simulink model "kinematics_crane"  (R2018b)
settings: Solver=VariableStepAuto  StartTime=0.0  StopTime=Tsim  RelTol=1e-6
model workspace: external: MATLAB File kran_DataFile.m (data not in the file)
undefined symbols (not defined in the file or in its folder): smiData, Ts, X, Y, Z
libraries: sm_lib x99, nesl_utility x28, simulink_extras x2
(part 1 of 3)
settings Model: Creator=Marko  LastModifiedBy=mandicluka
settings SFSimCC: SimCustomHeaderCode="#include \"../temp_cfiles/c_code.h\""  SimParseCustomCode=off
settings SFSimCC: SimUserSources=|
  | ../temp_cfiles/base.c
  | ../temp_cfiles/pulley.c
  | ../temp_cfiles//rot.c
  | ../temp_cfiles/trans1.c
  | ../temp_cfiles/trans2.c
settings SimscapeCC: SimscapeLogType=all  SimscapeLogSimulationStatistics=on  SimscapeLogLimitData=off
settings ExplorerConfigSet: InternalSimMechanicsExplorerSettings="<ExplorerConfiguration><canonicalview>planar_xy</canonicalview><AnimationSetting><BasePlaybackSpeed>1.0</BasePlaybackSpeed><PlaybackSpeedFactor>1.0</PlaybackSpeedFactor></AnimationSetting><TilePanel><TileInfo><Tiles Columns=\"1\" Count=\"1\" Rows=\"1\"><Column Weight=\"1\"/><Row Weight=\"1\"/><Tile Height=\"1\" Width=\"1\" X=\"0\" Y=\"0\"/></Tiles></TileInfo><SceneInfo><SceneViewer><BGColor><R>0.60000002384185791</R><G>0.60000002384185791</G><B>0.60000002384185791</B></BGColor><Camera><DoPerspective>off</DoPerspective><Position><X>10.1383469879859511</X><Y>3.51643315137439361</Y><Z>-1.36564695488922516</Z></Position><Center><X>1.28157942243814538</X><Y>3.51643315137439361</Y><Z>-1.36564695488922516</Z></Center><Up><X>0</X><Y>1</Y><Z>0</Z></Up><ViewLimDist>1</ViewLimDist><YLim>6.81084416950491534</YLim><XLim>4.8510498406429976</XLim></Camera></SceneViewer></SceneInfo></TilePanel><MechEditorPanel><Cameras/><GfxPanelCameraMap/><VideoCreator><PlaybackSpeedRatio>1.0</PlaybackSpeedRatio><FrameRate>30</FrameRate><VideoFormat>Motion JPEG AVI</VideoFormat><FrameSize>auto</FrameSize></VideoCreator></MechEditorPanel></ExplorerConfiguration>"

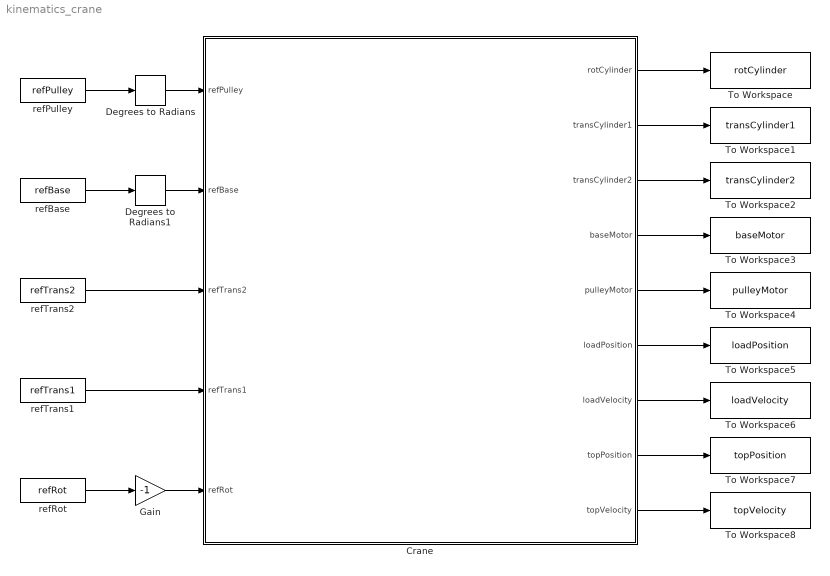
== system kinematics_crane ==
  Crane : Subsystem
  Degrees to Radians : simulink_extras/Transformations/Degrees to Radians
  Degrees to Radians1 : simulink_extras/Transformations/Degrees to Radians
  Gain : Gain  Gain=-1
  To Workspace : ToWorkspace  VariableName=rotCylinder  SaveFormat=Structure With Time  SampleTime=Ts
  To Workspace1 : ToWorkspace  VariableName=transCylinder1  SaveFormat=Structure With Time  SampleTime=Ts
  To Workspace2 : ToWorkspace  VariableName=transCylinder2  SaveFormat=Structure With Time  SampleTime=Ts
  To Workspace3 : ToWorkspace  VariableName=baseMotor  SaveFormat=Structure With Time  SampleTime=Ts
  To Workspace4 : ToWorkspace  VariableName=pulleyMotor  SaveFormat=Structure With Time  SampleTime=Ts
  To Workspace5 : ToWorkspace  VariableName=loadPosition  SaveFormat=Structure With Time  SampleTime=Ts
  To Workspace6 : ToWorkspace  VariableName=loadVelocity  SaveFormat=Structure With Time  SampleTime=Ts
  To Workspace7 : ToWorkspace  VariableName=topPosition  SaveFormat=Structure With Time  SampleTime=Ts
  To Workspace8 : ToWorkspace  VariableName=topVelocity  SaveFormat=Structure With Time  SampleTime=Ts
  refBase : FromWorkspace  VariableName=refBase  SampleTime=0  OutputAfterFinalValue=Holding final value
  refPulley : FromWorkspace  VariableName=refPulley  SampleTime=0  OutputAfterFinalValue=Holding final value
  refRot : FromWorkspace  VariableName=refRot  SampleTime=0  OutputAfterFinalValue=Holding final value
  refTrans1 : FromWorkspace  VariableName=refTrans1  SampleTime=0  OutputAfterFinalValue=Holding final value
  refTrans2 : FromWorkspace  VariableName=refTrans2  SampleTime=0  OutputAfterFinalValue=Holding final value
  wires:
  Crane/1(rotCylinder) -> To Workspace/1
  Crane/2(transCylinder1) -> To Workspace1/1
  Crane/3(transCylinder2) -> To Workspace2/1
  Crane/4(baseMotor) -> To Workspace3/1
  Crane/5(pulleyMotor) -> To Workspace4/1
  Crane/6(loadPosition) -> To Workspace5/1
  Crane/7(loadVelocity) -> To Workspace6/1
  Crane/8(topPosition) -> To Workspace7/1
  Crane/9(topVelocity) -> To Workspace8/1
  refPulley/1 -> Degrees to Radians/1
  refBase/1 -> Degrees to Radians1/1
  refTrans2/1 -> Crane/3(refTrans2)
  refTrans1/1 -> Crane/4(refTrans1)
  refRot/1 -> Gain/1
  Degrees to Radians/1 -> Crane/1(refPulley)
  Degrees to Radians1/1 -> Crane/2(refBase)
  Gain/1 -> Crane/5(refRot)

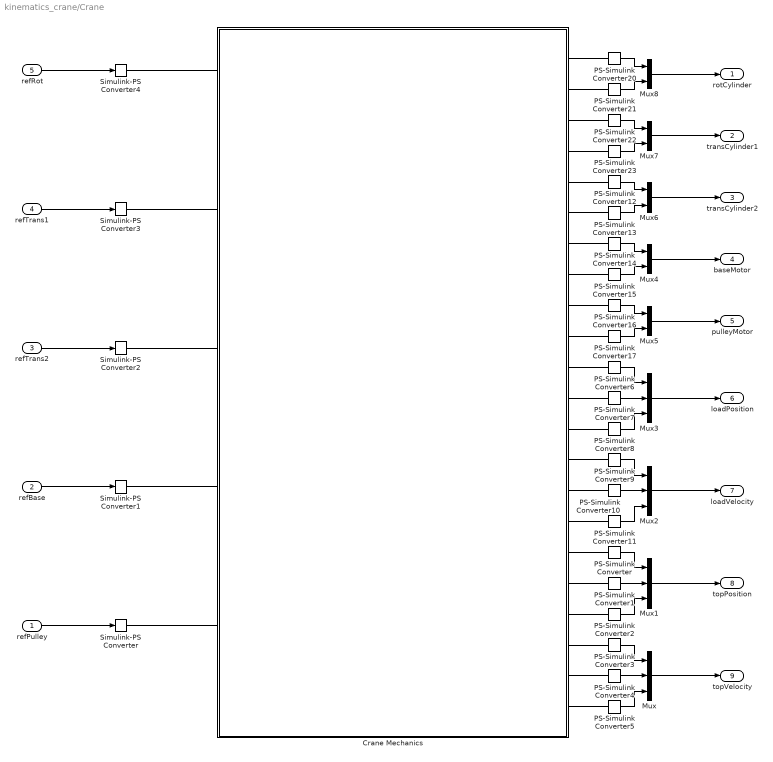
== system kinematics_crane/Crane ==
  refPulley : Inport
  refBase : Inport  Port=2
  refTrans2 : Inport  Port=3
  refTrans1 : Inport  Port=4
  refRot : Inport  Port=5
  Crane Mechanics : Subsystem
  Mux{,1..3} (4 alike) : Mux  Inputs=3
  Mux{4..8} (5 alike) : Mux  Inputs=2
  PS-Simulink Converter{,1..17,20..23} (22 alike) : nesl_utility/PS-Simulink Converter  PhysicalDomain=network_engine_domain  SubClassName=ps_output  LeftPortType=input  RightPortType=output  PseudoPeriodic=off  Frequencies=[]  Unit=1  AffineConversion=off
  Simulink-PS Converter{,1..4} (5 alike) : nesl_utility/Simulink-PS Converter  PhysicalDomain=network_engine_domain  SubClassName=ps_input  LeftPortType=input  RightPortType=output  PseudoPeriodic=off  Frequencies=[]  NoiseDistribution=none  NoiseParameters=[]  Unit=1  AffineConversion=off  FilteringAndDerivatives=filter  SimscapeFilterOrder=2  InputFilterTimeConstant=0.001  UdotUserProvided=0
  rotCylinder : Outport
  transCylinder1 : Outport  Port=2
  transCylinder2 : Outport  Port=3
  baseMotor : Outport  Port=4
  pulleyMotor : Outport  Port=5
  loadPosition : Outport  Port=6
  loadVelocity : Outport  Port=7
  topPosition : Outport  Port=8
  topVelocity : Outport  Port=9
  wires:
  PS-Simulink Converter12/1 -> Mux6/1
  Mux2/1 -> loadVelocity/1
  PS-Simulink Converter11/1 -> Mux2/3
  PS-Simulink Converter22/1 -> Mux7/1
  Mux3/1 -> loadPosition/1
  PS-Simulink Converter4/1 -> Mux/2
  PS-Simulink Converter17/1 -> Mux5/2
  PS-Simulink Converter15/1 -> Mux4/2
  PS-Simulink Converter1/1 -> Mux1/2
  PS-Simulink Converter/1 -> Mux1/1
  PS-Simulink Converter21/1 -> Mux8/2
  PS-Simulink Converter9/1 -> Mux2/1
  PS-Simulink Converter8/1 -> Mux3/3
  PS-Simulink Converter10/1 -> Mux2/2
  PS-Simulink Converter6/1 -> Mux3/1
  PS-Simulink Converter14/1 -> Mux4/1
  PS-Simulink Converter13/1 -> Mux6/2
  Mux6/1 -> transCylinder2/1
  PS-Simulink Converter16/1 -> Mux5/1
  PS-Simulink Converter3/1 -> Mux/1
  PS-Simulink Converter20/1 -> Mux8/1
  PS-Simulink Converter23/1 -> Mux7/2
  Mux1/1 -> topPosition/1
  PS-Simulink Converter5/1 -> Mux/3
  PS-Simulink Converter2/1 -> Mux1/3
  PS-Simulink Converter7/1 -> Mux3/2
  Mux7/1 -> transCylinder1/1
  Mux4/1 -> baseMotor/1
  Mux/1 -> topVelocity/1
  Mux5/1 -> pulleyMotor/1
  Mux8/1 -> rotCylinder/1
  refPulley/1 -> Simulink-PS Converter/1
  refBase/1 -> Simulink-PS Converter1/1
  refTrans2/1 -> Simulink-PS Converter2/1
  refTrans1/1 -> Simulink-PS Converter3/1
  refRot/1 -> Simulink-PS Converter4/1
  connections:
  Crane Mechanics/RConn5 -- PS-Simulink Converter12/LConn1
  Crane Mechanics/RConn7 -- PS-Simulink Converter14/LConn1
  Crane Mechanics/RConn14 -- PS-Simulink Converter9/LConn1
  Crane Mechanics/RConn6 -- PS-Simulink Converter13/LConn1
  Crane Mechanics/RConn15 -- PS-Simulink Converter10/LConn1
  Crane Mechanics/RConn9 -- PS-Simulink Converter16/LConn1
  PS-Simulink Converter2/LConn1 -- Crane Mechanics/RConn19
  Crane Mechanics/RConn16 -- PS-Simulink Converter11/LConn1
  Crane Mechanics/RConn11 -- PS-Simulink Converter6/LConn1
  PS-Simulink Converter5/LConn1 -- Crane Mechanics/RConn22
  Crane Mechanics/RConn4 -- PS-Simulink Converter23/LConn1
  Crane Mechanics/RConn13 -- PS-Simulink Converter8/LConn1
  PS-Simulink Converter/LConn1 -- Crane Mechanics/RConn17
  Crane Mechanics/RConn3 -- PS-Simulink Converter22/LConn1
  Crane Mechanics/RConn8 -- PS-Simulink Converter15/LConn1
  PS-Simulink Converter4/LConn1 -- Crane Mechanics/RConn21
  Crane Mechanics/RConn2 -- PS-Simulink Converter21/LConn1
  Crane Mechanics/RConn12 -- PS-Simulink Converter7/LConn1
  Crane Mechanics/RConn1 -- PS-Simulink Converter20/LConn1
  PS-Simulink Converter1/LConn1 -- Crane Mechanics/RConn18
  Crane Mechanics/RConn10 -- PS-Simulink Converter17/LConn1
  PS-Simulink Converter3/LConn1 -- Crane Mechanics/RConn20
  Simulink-PS Converter/RConn1 -- Crane Mechanics/LConn9
  Crane Mechanics/LConn7 -- Simulink-PS Converter1/RConn1
  Crane Mechanics/LConn5 -- Simulink-PS Converter2/RConn1
  Crane Mechanics/LConn3 -- Simulink-PS Converter3/RConn1
  Crane Mechanics/LConn1 -- Simulink-PS Converter4/RConn1

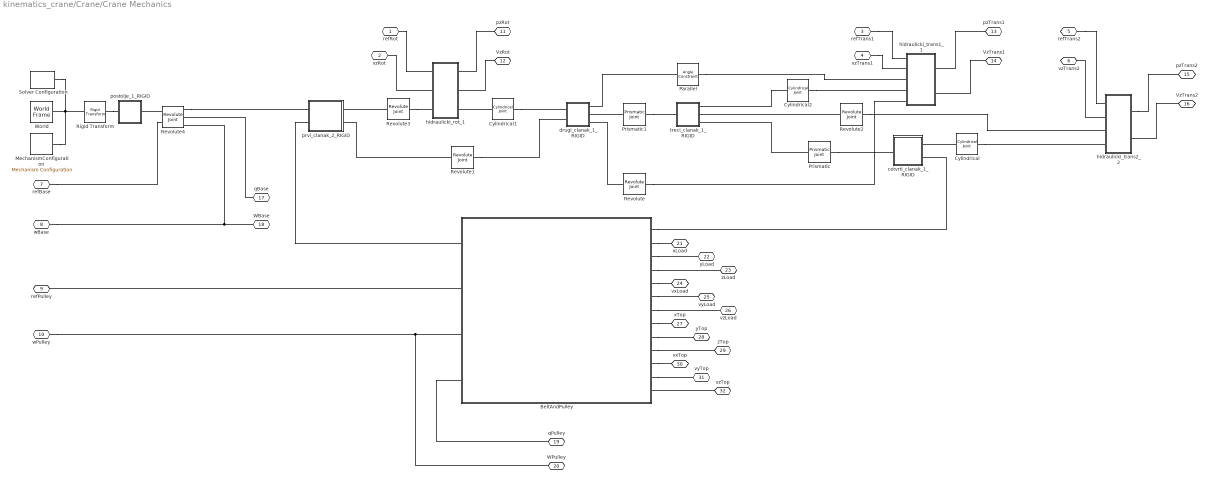
== system kinematics_crane/Crane/Crane Mechanics ==
  BeltAndPulley : Subsystem
  Cylindrical : sm_lib/Joints/Cylindrical Joint  SenseConstraintForce=off  SenseConstraintForceX=off  SenseConstraintForceY=off  SenseConstraintForceZ=off  SenseConstraintTorque=off  SenseConstraintTorqueX=off  SenseConstraintTorqueY=off  SenseConstraintTorqueZ=off  SenseTotalForce=off  SenseTotalForceX=off  SenseTotalForceY=off  SenseTotalForceZ=off  SenseTotalTorque=off  SenseTotalTorqueX=off  SenseTotalTorqueY=off  SenseTotalTorqueZ=off  CompositeWrenchDir=FollowerOnBase  CompositeWrenchFrame=BaseFrame  PzEquilibriumPosition=0  PzEquilibriumPositionUnits=m  PzSpringStiffness=0  PzSpringStiffnessUnits=N/m  PzDampingCoefficient=0  PzDampingCoefficientUnits=N/(m/s)  PzTorqueActuationMode=NoTorque  PzMotionActuationMode=ComputedMotion  PzSensePosition=off  PzSenseVelocity=off  PzSenseAcceleration=off  PzSenseTorqueForce=off  PzPositionTargetSpecify=off  PzPositionTargetPriority=High  PzPositionTargetValue=0  PzPositionTargetValueUnits=m  PzVelocityTargetSpecify=off  PzVelocityTargetPriority=High  PzVelocityTargetValue=0  PzVelocityTargetValueUnits=m/s  RzEquilibriumPosition=0  RzEquilibriumPositionUnits=rad  RzSpringStiffness=0  RzSpringStiffnessUnits=N*m/rad  RzDampingCoefficient=0  RzDampingCoefficientUnits=N*m/(rad/s)  RzTorqueActuationMode=NoTorque  RzMotionActuationMode=ComputedMotion  RzSensePosition=off  RzSenseVelocity=off  RzSenseAcceleration=off  RzSenseTorqueForce=off  RzPositionTargetSpecify=off  RzPositionTargetPriority=High  RzPositionTargetValue=0  RzPositionTargetValueUnits=deg  RzVelocityTargetSpecify=off  RzVelocityTargetPriority=High  RzVelocityTargetValue=0  RzVelocityTargetValueUnits=deg/s
  Cylindrical1 : sm_lib/Joints/Cylindrical Joint  SenseConstraintForce=off  SenseConstraintForceX=off  SenseConstraintForceY=off  SenseConstraintForceZ=off  SenseConstraintTorque=off  SenseConstraintTorqueX=off  SenseConstraintTorqueY=off  SenseConstraintTorqueZ=off  SenseTotalForce=off  SenseTotalForceX=off  SenseTotalForceY=off  SenseTotalForceZ=off  SenseTotalTorque=off  SenseTotalTorqueX=off  SenseTotalTorqueY=off  SenseTotalTorqueZ=off  CompositeWrenchDir=FollowerOnBase  CompositeWrenchFrame=BaseFrame  PzEquilibriumPosition=0  PzEquilibriumPositionUnits=m  PzSpringStiffness=0  PzSpringStiffnessUnits=N/m  PzDampingCoefficient=0  PzDampingCoefficientUnits=N/(m/s)  PzTorqueActuationMode=NoTorque  PzMotionActuationMode=ComputedMotion  PzSensePosition=off  PzSenseVelocity=off  PzSenseAcceleration=off  PzSenseTorqueForce=off  PzPositionTargetSpecify=off  PzPositionTargetPriority=High  PzPositionTargetValue=0  PzPositionTargetValueUnits=m  PzVelocityTargetSpecify=off  PzVelocityTargetPriority=High  PzVelocityTargetValue=0  PzVelocityTargetValueUnits=m/s  RzEquilibriumPosition=0  RzEquilibriumPositionUnits=rad  RzSpringStiffness=0  RzSpringStiffnessUnits=N*m/rad  RzDampingCoefficient=0  RzDampingCoefficientUnits=N*m/(rad/s)  RzTorqueActuationMode=NoTorque  RzMotionActuationMode=ComputedMotion  RzSensePosition=off  RzSenseVelocity=off  RzSenseAcceleration=off  RzSenseTorqueForce=off  RzPositionTargetSpecify=off  RzPositionTargetPriority=High  RzPositionTargetValue=0  RzPositionTargetValueUnits=deg  RzVelocityTargetSpecify=off  RzVelocityTargetPriority=High  RzVelocityTargetValue=0  RzVelocityTargetValueUnits=deg/s
  Cylindrical2 : sm_lib/Joints/Cylindrical Joint  SenseConstraintForce=off  SenseConstraintForceX=off  SenseConstraintForceY=off  SenseConstraintForceZ=off  SenseConstraintTorque=off  SenseConstraintTorqueX=off  SenseConstraintTorqueY=off  SenseConstraintTorqueZ=off  SenseTotalForce=off  SenseTotalForceX=off  SenseTotalForceY=off  SenseTotalForceZ=off  SenseTotalTorque=off  SenseTotalTorqueX=off  SenseTotalTorqueY=off  SenseTotalTorqueZ=off  CompositeWrenchDir=FollowerOnBase  CompositeWrenchFrame=BaseFrame  PzEquilibriumPosition=0  PzEquilibriumPositionUnits=m  PzSpringStiffness=0  PzSpringStiffnessUnits=N/m  PzDampingCoefficient=0  PzDampingCoefficientUnits=N/(m/s)  PzTorqueActuationMode=NoTorque  PzMotionActuationMode=ComputedMotion  PzSensePosition=off  PzSenseVelocity=off  PzSenseAcceleration=off  PzSenseTorqueForce=off  PzPositionTargetSpecify=off  PzPositionTargetPriority=High  PzPositionTargetValue=0  PzPositionTargetValueUnits=m  PzVelocityTargetSpecify=off  PzVelocityTargetPriority=High  PzVelocityTargetValue=0  PzVelocityTargetValueUnits=m/s  RzEquilibriumPosition=0  RzEquilibriumPositionUnits=rad  RzSpringStiffness=0  RzSpringStiffnessUnits=N*m/rad  RzDampingCoefficient=0  RzDampingCoefficientUnits=N*m/(rad/s)  RzTorqueActuationMode=NoTorque  RzMotionActuationMode=ComputedMotion  RzSensePosition=off  RzSenseVelocity=off  RzSenseAcceleration=off  RzSenseTorqueForce=off  RzPositionTargetSpecify=off  RzPositionTargetPriority=High  RzPositionTargetValue=0  RzPositionTargetValueUnits=deg  RzVelocityTargetSpecify=off  RzVelocityTargetPriority=High  RzVelocityTargetValue=0  RzVelocityTargetValueUnits=deg/s
  MechanismConfiguration : sm_lib/Utilities/Mechanism Configuration  UniformGravity=Constant  GravityVector=[0 -9.80665 0]  GravityUnits=m/s^2  LinearizationDelta=0.001
  Parallel : sm_lib/Constraints/Angle Constraint  ConstraintType=Parallel  Angle=45  AngleUnits=deg  SenseSignedTorqueMagnitude=off  SenseTorque=off  SenseForce=off  WrenchDir=FollowerOnBase  WrenchFrame=BaseFrame
      settings: SourceProductName=Simscape Multibody  SourceProductBaseCode=MS
  Prismatic : sm_lib/Joints/Prismatic Joint  SenseConstraintForce=off  SenseConstraintForceX=off  SenseConstraintForceY=off  SenseConstraintForceZ=off  SenseConstraintTorque=off  SenseConstraintTorqueX=off  SenseConstraintTorqueY=off  SenseConstraintTorqueZ=off  SenseTotalForce=off  SenseTotalForceX=off  SenseTotalForceY=off  SenseTotalForceZ=off  SenseTotalTorque=off  SenseTotalTorqueX=off  SenseTotalTorqueY=off  SenseTotalTorqueZ=off  CompositeWrenchDir=FollowerOnBase  CompositeWrenchFrame=BaseFrame  EquilibriumPosition=0  EquilibriumPositionUnits=m  SpringStiffness=0  SpringStiffnessUnits=N/m  DampingCoefficient=0  DampingCoefficientUnits=N/(m/s)  TorqueActuationMode=NoTorque  MotionActuationMode=ComputedMotion  SensePosition=off  SenseVelocity=off  SenseAcceleration=off  SenseTorqueForce=off  PositionTargetSpecify=on  PositionTargetPriority=Low  PositionTargetValue=smiData.PrismaticJoint(1).Pz.Pos  PositionTargetValueUnits=m  VelocityTargetSpecify=off  VelocityTargetPriority=High  VelocityTargetValue=0  VelocityTargetValueUnits=m/s
  Prismatic1 : sm_lib/Joints/Prismatic Joint  SenseConstraintForce=off  SenseConstraintForceX=off  SenseConstraintForceY=off  SenseConstraintForceZ=off  SenseConstraintTorque=off  SenseConstraintTorqueX=off  SenseConstraintTorqueY=off  SenseConstraintTorqueZ=off  SenseTotalForce=off  SenseTotalForceX=off  SenseTotalForceY=off  SenseTotalForceZ=off  SenseTotalTorque=off  SenseTotalTorqueX=off  SenseTotalTorqueY=off  SenseTotalTorqueZ=off  CompositeWrenchDir=FollowerOnBase  CompositeWrenchFrame=BaseFrame  EquilibriumPosition=0  EquilibriumPositionUnits=m  SpringStiffness=0  SpringStiffnessUnits=N/m  DampingCoefficient=0  DampingCoefficientUnits=N/(m/s)  TorqueActuationMode=NoTorque  MotionActuationMode=ComputedMotion  SensePosition=off  SenseVelocity=off  SenseAcceleration=off  SenseTorqueForce=off  PositionTargetSpecify=on  PositionTargetPriority=Low  PositionTargetValue=smiData.PrismaticJoint(2).Pz.Pos  PositionTargetValueUnits=m  VelocityTargetSpecify=off  VelocityTargetPriority=High  VelocityTargetValue=0  VelocityTargetValueUnits=m/s
  Revolute : sm_lib/Joints/Revolute Joint  SenseConstraintForce=off  SenseConstraintForceX=off  SenseConstraintForceY=off  SenseConstraintForceZ=off  SenseConstraintTorque=off  SenseConstraintTorqueX=off  SenseConstraintTorqueY=off  SenseConstraintTorqueZ=off  SenseTotalForce=off  SenseTotalForceX=off  SenseTotalForceY=off  SenseTotalForceZ=off  SenseTotalTorque=off  SenseTotalTorqueX=off  SenseTotalTorqueY=off  SenseTotalTorqueZ=off  CompositeWrenchDir=FollowerOnBase  CompositeWrenchFrame=BaseFrame  EquilibriumPosition=0  EquilibriumPositionUnits=rad  SpringStiffness=0  SpringStiffnessUnits=N*m/rad  DampingCoefficient=0  DampingCoefficientUnits=N*m/(rad/s)  TorqueActuationMode=NoTorque  MotionActuationMode=ComputedMotion  SensePosition=off  SenseVelocity=off  SenseAcceleration=off  SenseTorqueForce=off  PositionTargetSpecify=on  PositionTargetPriority=Low  PositionTargetValue=smiData.RevoluteJoint(4).Rz.Pos  PositionTargetValueUnits=deg  VelocityTargetSpecify=off  VelocityTargetPriority=High  VelocityTargetValue=0  VelocityTargetValueUnits=deg/s
  Revolute1 : sm_lib/Joints/Revolute Joint  SenseConstraintForce=off  SenseConstraintForceX=off  SenseConstraintForceY=off  SenseConstraintForceZ=off  SenseConstraintTorque=off  SenseConstraintTorqueX=off  SenseConstraintTorqueY=off  SenseConstraintTorqueZ=off  SenseTotalForce=off  SenseTotalForceX=off  SenseTotalForceY=off  SenseTotalForceZ=off  SenseTotalTorque=off  SenseTotalTorqueX=off  SenseTotalTorqueY=off  SenseTotalTorqueZ=off  CompositeWrenchDir=FollowerOnBase  CompositeWrenchFrame=BaseFrame  EquilibriumPosition=0  EquilibriumPositionUnits=rad  SpringStiffness=0  SpringStiffnessUnits=N*m/rad  DampingCoefficient=0  DampingCoefficientUnits=N*m/(rad/s)  TorqueActuationMode=NoTorque  MotionActuationMode=ComputedMotion  SensePosition=off  SenseVelocity=off  SenseAcceleration=off  SenseTorqueForce=off  PositionTargetSpecify=on  PositionTargetPriority=Low  PositionTargetValue=smiData.RevoluteJoint(5).Rz.Pos  PositionTargetValueUnits=deg  VelocityTargetSpecify=off  VelocityTargetPriority=High  VelocityTargetValue=0  VelocityTargetValueUnits=deg/s
  Revolute2 : sm_lib/Joints/Revolute Joint  SenseConstraintForce=off  SenseConstraintForceX=off  SenseConstraintForceY=off  SenseConstraintForceZ=off  SenseConstraintTorque=off  SenseConstraintTorqueX=off  SenseConstraintTorqueY=off  SenseConstraintTorqueZ=off  SenseTotalForce=off  SenseTotalForceX=off  SenseTotalForceY=off  SenseTotalForceZ=off  SenseTotalTorque=off  SenseTotalTorqueX=off  SenseTotalTorqueY=off  SenseTotalTorqueZ=off  CompositeWrenchDir=FollowerOnBase  CompositeWrenchFrame=BaseFrame  EquilibriumPosition=0  EquilibriumPositionUnits=rad  SpringStiffness=0  SpringStiffnessUnits=N*m/rad  DampingCoefficient=0  DampingCoefficientUnits=N*m/(rad/s)  TorqueActuationMode=NoTorque  MotionActuationMode=ComputedMotion  SensePosition=off  SenseVelocity=off  SenseAcceleration=off  SenseTorqueForce=off  PositionTargetSpecify=on  PositionTargetPriority=Low  PositionTargetValue=smiData.RevoluteJoint(6).Rz.Pos  PositionTargetValueUnits=deg  VelocityTargetSpecify=off  VelocityTargetPriority=High  VelocityTargetValue=0  VelocityTargetValueUnits=deg/s
  Revolute3 : sm_lib/Joints/Revolute Joint  SenseConstraintForce=off  SenseConstraintForceX=off  SenseConstraintForceY=off  SenseConstraintForceZ=off  SenseConstraintTorque=off  SenseConstraintTorqueX=off  SenseConstraintTorqueY=off  SenseConstraintTorqueZ=off  SenseTotalForce=off  SenseTotalForceX=off  SenseTotalForceY=off  SenseTotalForceZ=off  SenseTotalTorque=off  SenseTotalTorqueX=off  SenseTotalTorqueY=off  SenseTotalTorqueZ=off  CompositeWrenchDir=FollowerOnBase  CompositeWrenchFrame=BaseFrame  EquilibriumPosition=0  EquilibriumPositionUnits=rad  SpringStiffness=0  SpringStiffnessUnits=N*m/rad  DampingCoefficient=0  DampingCoefficientUnits=N*m/(rad/s)  TorqueActuationMode=NoTorque  MotionActuationMode=ComputedMotion  SensePosition=off  SenseVelocity=off  SenseAcceleration=off  SenseTorqueForce=off  PositionTargetSpecify=on  PositionTargetPriority=Low  PositionTargetValue=smiData.RevoluteJoint(7).Rz.Pos  PositionTargetValueUnits=deg  VelocityTargetSpecify=off  VelocityTargetPriority=High  VelocityTargetValue=0  VelocityTargetValueUnits=deg/s
  Revolute4 : sm_lib/Joints/Revolute Joint  SenseConstraintForce=off  SenseConstraintForceX=off  SenseConstraintForceY=off  SenseConstraintForceZ=off  SenseConstraintTorque=off  SenseConstraintTorqueX=off  SenseConstraintTorqueY=off  SenseConstraintTorqueZ=off  SenseTotalForce=off  SenseTotalForceX=off  SenseTotalForceY=off  SenseTotalForceZ=off  SenseTotalTorque=off  SenseTotalTorqueX=off  SenseTotalTorqueY=off  SenseTotalTorqueZ=off  CompositeWrenchDir=FollowerOnBase  CompositeWrenchFrame=BaseFrame  EquilibriumPosition=0  EquilibriumPositionUnits=rad  SpringStiffness=0  SpringStiffnessUnits=N*m/rad  DampingCoefficient=500  DampingCoefficientUnits=N*m/(rad/s)  TorqueActuationMode=ComputedTorque  MotionActuationMode=InputMotion  SensePosition=on  SenseVelocity=on  SenseAcceleration=off  SenseTorqueForce=off  PositionTargetSpecify=on  PositionTargetPriority=High  PositionTargetValue=0  PositionTargetValueUnits=deg  VelocityTargetSpecify=off  VelocityTargetPriority=High  VelocityTargetValue=0  VelocityTargetValueUnits=deg/s
  Rigid Transform : sm_lib/Frames and Transforms/Rigid Transform  TranslationMethod=Cartesian  TranslationStandardOffset=0  TranslationLengthUnit=m  TranslationStandardAxis=+Z  TranslationCartesianOffset=[0 0.86 0]  TranslationROffset=0  TranslationROffsetUnits=m  TranslationZOffset=0  TranslationZOffsetUnits=m  TranslationThetaOffset=0  TranslationThetaOffsetUnits=deg  RotationMethod=StandardAxis  RotationAngleUnits=deg  RotationStandardAxis=-Y  RotationAngle=90  RotationArbitraryAxis=[0 0 1]  FollAlignAxisA=+X  BaseAlignAxisA=+Y  FollAlignAxisB=+Y  BaseAlignAxisB=+Z  RotationSequenceAxes=FollowerAxes  RotationSequence=XYX  RotationSequenceAngles=[0 0 0]  RotationSequenceAnglesUnits=deg  RotationMatrix=[1 0 0; 0 1 0; 0 0 1]
  Solver Configuration : nesl_utility/Solver Configuration  PhysicalDomain=network_engine_domain  SubClassName=solver  LeftPortType=input  RightPortType=generic  Tones=[]  Harmonics=[]  SimulateNoise=off  Profile=off  UseLocalSampling=off  EnableSwitchedLinearOptims=on  FrequencyDomain=off  UseCCode=off  RelTol=0.001  AbsTol=1e-06  MinStep=1e-09  ToWorkspace=off  RevertToSquareIcSolve=off  NumHomotopyIterations=100  PhasorMode=off  PhasorModeNumHarmonics=1  DoDC=off  ResidualTolerance=1e-09  UseLocalSolver=off  LocalSolverChoice=NE_BACKWARD_EULER_ADVANCER  LocalSolverSampleTime=0.001  DoFixedCost=off  MaxNonlinIter=3  MaxModeIter=2  LinearAlgebra=auto  EquationFormulation=NE_TIME_EF  DelaysMemoryBudget=1024  AutomaticFiltering=on  FilteringTimeConstant=0.0001  PartitionStorageMethod=AS_NEEDED  PartitionMemoryBudget=1024
  World : sm_lib/Frames and Transforms/World Frame
  cetvrti_clanak_1_RIGID : Subsystem
  drugi_clanak_1_RIGID : Subsystem
  hidraulicki_rot_1 : Subsystem
  hidraulicki_trans1_1 : Subsystem
  hidraulicki_trans2_2 : Subsystem
  postolje_1_RIGID : Subsystem
  prvi_clanak_2_RIGID : Subsystem
  treci_clanak_1_RIGID : Subsystem
  refRot : PMIOPort  Side=Left
  vzRot : PMIOPort  Port=2  Side=Left
  refTrans1 : PMIOPort  Port=3  Side=Left
  vzTrans1 : PMIOPort  Port=4  Side=Left
  refTrans2 : PMIOPort  Port=5  Side=Left
  vzTrans2 : PMIOPort  Port=6  Side=Left
  refBase : PMIOPort  Port=7  Side=Left
  wBase : PMIOPort  Port=8  Side=Left
  refPulley : PMIOPort  Port=9  Side=Left
  wPulley : PMIOPort  Port=10  Side=Left
  pzRot : PMIOPort  Port=11  Side=Right
  VzRot : PMIOPort  Port=12  Side=Right
  pzTrans1 : PMIOPort  Port=13  Side=Right
  VzTrans1 : PMIOPort  Port=14  Side=Right
  pzTrans2 : PMIOPort  Port=15  Side=Right
  VzTrans2 : PMIOPort  Port=16  Side=Right
  qBase : PMIOPort  Port=17  Side=Right
  WBase : PMIOPort  Port=18  Side=Right
  qPulley : PMIOPort  Port=19  Side=Right
  WPulley : PMIOPort  Port=20  Side=Right
  xLoad : PMIOPort  Port=21  Side=Right
  yLoad : PMIOPort  Port=22  Side=Right
  zLoad : PMIOPort  Port=23  Side=Right
  vxLoad : PMIOPort  Port=24  Side=Right
  vyLoad : PMIOPort  Port=25  Side=Right
  vzLoad : PMIOPort  Port=26  Side=Right
  xTop : PMIOPort  Port=27  Side=Right
  yTop : PMIOPort  Port=28  Side=Right
  zTop : PMIOPort  Port=29  Side=Right
  vxTop : PMIOPort  Port=30  Side=Right
  vyTop : PMIOPort  Port=31  Side=Right
  vzTop : PMIOPort  Port=32  Side=Right
  connections:
  Cylindrical2/RConn1 -- hidraulicki_trans1_1/LConn4
  MechanismConfiguration/RConn1 -- Solver Configuration/RConn1 -- World/RConn1 -- Rigid Transform/LConn1
  Revolute4/LConn1 -- postolje_1_RIGID/RConn1
  Revolute1/LConn1 -- prvi_clanak_2_RIGID/RConn2
  Revolute2/RConn1 -- hidraulicki_trans2_2/LConn3
  Revolute4/RConn1 -- prvi_clanak_2_RIGID/LConn1
  Cylindrical1/LConn1 -- hidraulicki_rot_1/RConn3
  Parallel/LConn1 -- drugi_clanak_1_RIGID/RConn1
  Revolute3/LConn1 -- prvi_clanak_2_RIGID/RConn1
  Prismatic/LConn1 -- treci_clanak_1_RIGID/RConn3
  Cylindrical1/RConn1 -- drugi_clanak_1_RIGID/LConn1
  Prismatic/RConn1 -- cetvrti_clanak_1_RIGID/LConn1
  Cylindrical2/LConn1 -- treci_clanak_1_RIGID/RConn1
  Revolute/LConn1 -- drugi_clanak_1_RIGID/RConn3
  Parallel/RConn1 -- hidraulicki_trans1_1/LConn3
  Revolute1/RConn1 -- drugi_clanak_1_RIGID/LConn2
  Prismatic1/LConn1 -- drugi_clanak_1_RIGID/RConn2
  Cylindrical/RConn1 -- hidraulicki_trans2_2/LConn4
  Revolute3/RConn1 -- hidraulicki_rot_1/LConn3
  Revolute/RConn1 -- hidraulicki_trans1_1/LConn5
  Prismatic1/RConn1 -- treci_clanak_1_RIGID/LConn1
  Cylindrical/LConn1 -- cetvrti_clanak_1_RIGID/RConn1
  Revolute2/LConn1 -- treci_clanak_1_RIGID/RConn2
  hidraulicki_rot_1/LConn2 -- vzRot/RConn1
  refRot/RConn1 -- hidraulicki_rot_1/LConn1
  refTrans1/RConn1 -- hidraulicki_trans1_1/LConn1
  vzTrans1/RConn1 -- hidraulicki_trans1_1/LConn2
  refTrans2/RConn1 -- hidraulicki_trans2_2/LConn1
  hidraulicki_trans2_2/LConn2 -- vzTrans2/RConn1
  prvi_clanak_2_RIGID/LConn2 -- BeltAndPulley/LConn1
  BeltAndPulley/RConn1 -- cetvrti_clanak_1_RIGID/RConn2
  BeltAndPulley/LConn2 -- refPulley/RConn1
  refBase/RConn1 -- Revolute4/LConn2
  wPulley/RConn1 -- WPulley/RConn1 -- BeltAndPulley/LConn3
  pzRot/RConn1 -- hidraulicki_rot_1/RConn1
  VzRot/RConn1 -- hidraulicki_rot_1/RConn2
  VzTrans1/RConn1 -- hidraulicki_trans1_1/RConn2
  pzTrans1/RConn1 -- hidraulicki_trans1_1/RConn1
  VzTrans2/RConn1 -- hidraulicki_trans2_2/RConn2
  hidraulicki_trans2_2/RConn1 -- pzTrans2/RConn1
  wBase/RConn1 -- WBase/RConn1 -- Revolute4/RConn3
  qBase/RConn1 -- Revolute4/RConn2
  qPulley/RConn1 -- BeltAndPulley/LConn4
  BeltAndPulley/RConn2 -- xLoad/RConn1
  BeltAndPulley/RConn3 -- yLoad/RConn1
  BeltAndPulley/RConn4 -- zLoad/RConn1
  BeltAndPulley/RConn5 -- vxLoad/RConn1
  BeltAndPulley/RConn6 -- vyLoad/RConn1
  BeltAndPulley/RConn7 -- vzLoad/RConn1
  BeltAndPulley/RConn12 -- vyTop/RConn1
  BeltAndPulley/RConn11 -- vxTop/RConn1
  BeltAndPulley/RConn10 -- zTop/RConn1
  BeltAndPulley/RConn8 -- xTop/RConn1
  BeltAndPulley/RConn9 -- yTop/RConn1
  vzTop/RConn1 -- BeltAndPulley/RConn13
  Rigid Transform/RConn1 -- postolje_1_RIGID/LConn1
